simulink model "GraneBaseModel"  (R2017b)
settings: Solver=FixedStepAuto  StartTime=0.0  StopTime=10  FixedStep=0.01  RelTol=1e-3
undefined symbols (not defined in the file or in its folder): National_Instruments, PCI
libraries: sldrtlib x4
settings Model: Creator=labadmin  LastModifiedBy=labadmin
settings RTWCC: SystemTargetFile=sldrt.tlc  TemplateMakefile=sldrt.tmf  Description=Simulink Desktop Real-Time  RTWCompilerOptimization=on
settings CodeAppCC: MaxIdLength=95
settings SimulinkDesktopRealTimeCC: TargetPreCompLibLocation=C:\Program Files\MATLAB\R2017b\toolbox\sldrt\lib\win64

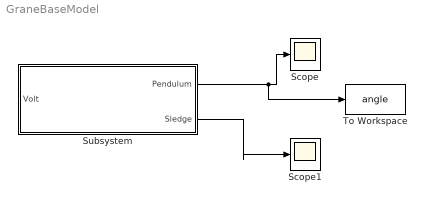
== system GraneBaseModel ==
  Scope : Scope
  Scope1 : Scope
  Subsystem : Subsystem
  To Workspace : ToWorkspace  VariableName=angle  SaveFormat=Timeseries  SampleTime=-1
  wires:
  Subsystem/1(Pendulum) -> To Workspace/1, Scope/1
  Subsystem/2(Sledge) -> Scope1/1

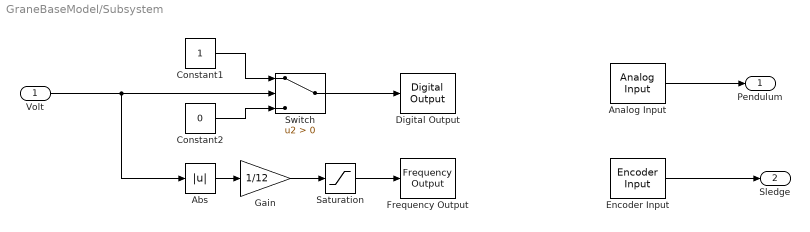
== system GraneBaseModel/Subsystem ==
  Volt : Inport
  Abs : Abs
  Analog Input : sldrtlib/Analog Input  SampleTime=-1  MaxMissedTicks=1000000000  ShowMissedTicks=off  YieldWhenWaiting=off  DrvName=National_Instruments/PCI-6229  DrvAddress=4294967295  DrvOptions=[0 1 8192 2 3]  Channels=1  RangeMode=1  VoltRange=1  DataType=1
      settings: AttributesFormatString=National Instruments\nPCI-6229 [auto]  SourceProductName=Simulink Desktop Real-Time
  Constant1 : Constant
  Constant2 : Constant  Value=0
  Digital Output : sldrtlib/Digital Output  SampleTime=-1  MaxMissedTicks=100000000  ShowMissedTicks=off  YieldWhenWaiting=off  DrvName=National_Instruments/PCI-6229  DrvAddress=4294967295  DrvOptions=[0 1 8192 2 3]  Channels=1  BitMode=1  InitialValue=[]  FinalValue=[]
      settings: AttributesFormatString=National Instruments\nPCI-6229 [auto]  SourceProductName=Simulink Desktop Real-Time  SourceProductBaseCode=WT
  Encoder Input : sldrtlib/Encoder Input  SampleTime=-1  MaxMissedTicks=10000000  ShowMissedTicks=off  YieldWhenWaiting=off  DrvName=National_Instruments/PCI-6229  DrvAddress=4294967295  DrvOptions=[0 1 8192 2 3]  Channels=1  QuadMode=3  IndexPulse=2  InputFilter=Inf  DataType=1
      settings: AttributesFormatString=National Instruments\nPCI-6229 [auto]  SourceProductName=Simulink Desktop Real-Time
  Frequency Output : sldrtlib/Frequency Output  SampleTime=-1  MaxMissedTicks=1000000000  ShowMissedTicks=off  YieldWhenWaiting=off  DrvName=National_Instruments/PCI-6229  DrvAddress=4294967295  DrvOptions=[0 1 8192 2 3]  Channels=2  FrequencySource=1  Frequency=10000  FrequencyFinalValue=[]  DutySource=2  Duty=0  DutyFinalValue=0
      settings: AttributesFormatString=National Instruments\nPCI-6229 [auto]  SourceProductName=Simulink Desktop Real-Time  SourceProductBaseCode=WT
  Gain : Gain  Gain=1/12
  Saturation : Saturate  UpperLimit=0.35  LowerLimit=0
  Switch : Switch  Criteria=u2 > Threshold
  Pendulum : Outport
  Sledge : Outport  Port=2
  wires:
  Analog Input/1 -> Pendulum/1
  Encoder Input/1 -> Sledge/1
  Saturation/1 -> Frequency Output/1
  Volt/1 -> Abs/1, Switch/2
  Gain/1 -> Saturation/1
  Constant2/1 -> Switch/3
  Abs/1 -> Gain/1
  Constant1/1 -> Switch/1
  Switch/1 -> Digital Output/1
